simulink model "smm_with_grf_tilting_2d"  (R2014b)
settings: Solver=FixedStepDiscrete  StartTime=0.0  StopTime=inf  FixedStep=sample_time  RelTol=1e-3
undefined symbols (not defined in the file or in its folder): A_lpf_dtau, A_lpf_leg_spring, alpha_apex, alpha_max, alpha_min, B1_lpf_dtau, B1_lpf_leg_spring, B2_lpf_dtau, B2_lpf_leg_spring, boom_mount_angle, boom_pelvis_offset_angle, c_energy, contact_threshold, control_start_time, d_y_boom_com_offset, d_y_boom_hip_offset, d_y_com, desired_torso_angle, dx_avg_desired, enable_torso_wave, fcut_contact, ff_energy_l, ff_energy_r, g, g_reduced, h_boom, HIP_MTR_MAX_CONT_TORQUE, i_robot, initial_com_height, initial_dx, j_leg, j_motor, j_rotor, j_segments, k0_virtual, k_placement, k_sea, kd_lateral, kd_motor, kd_torso, kp_lateral, kp_motor, kp_raibert, kp_torso, l0_leg, l0_min_flight_time, l0_virtual, l0_virtual_raibert, l_boom_projected, l_max, l_retract_delta, l_retract_swing_max, l_retract_swing_min, l_seg, l_yaw_center_to_pelvis, lambda1, lambda2, lateral_offset, lateral_target_angle_left, lateral_target_angle_right ... (+40)
libraries: simulink x24, slrtlib x4, simulink_extras x2
(part 3 of 4)

== system smm_with_grf_tilting_2d/Control/Behavior Control/Primary Leg Behavior/SMM 01/Primary Swing Phase/Back//Front Motor PD ==
  Desired Position [rad] [back front] : Inport
  Desired Velocity [rad/s] [back front] : Inport  Port=2
  Desired Acceleration [rad/s^2] [back front] : Inport  Port=3
  Measured Position [rad] [back front] : Inport  Port=4
  Measured Velocity [rad/s] [back front] : Inport  Port=5
  Right/Left Leg [1/0] : Inport  Port=6
  Friction Compensation : Subsystem
  Product : Product
  Sum1 : Sum  Inputs=|++
  Sum2 : Sum  Inputs=|++
  Sum7 : Sum  Inputs=|+-
  Sum8 : Sum  Inputs=|+-
  Sum9 : Sum
  Switch : Switch  Criteria=u2 ~= 0
  kd : Gain  Gain=kd_motor
  kp : Gain  Gain=kp_motor
  left_inertias : Constant  Value=j_segments(3:4)
  right_inertias : Constant  Value=j_segments(1:2)
  Commanded Torque [Nm] [back front] : Outport
  wires:
  kp/1 -> Sum9/1
  Sum7/1 -> kp/1
  Measured Position [rad] [back front]/1 -> Sum7/2
  Sum9/1 -> Sum1/1
  Sum8/1 -> kd/1
  Desired Position [rad] [back front]/1 -> Sum7/1
  kd/1 -> Sum9/2
  Measured Velocity [rad/s] [back front]/1 -> Sum8/2
  Sum1/1 -> Sum2/1
  Desired Acceleration [rad/s^2] [back front]/1 -> Product/1
  Product/1 -> Sum1/2
  Right/Left Leg [1/0]/1 -> Friction Compensation/1(Right/Left [1/0]), Switch/2
  right_inertias/1 -> Switch/1
  left_inertias/1 -> Switch/3
  Switch/1 -> Product/2
  Sum2/1 -> Commanded Torque [Nm] [back front]/1
  Friction Compensation/1(Friction Compensation [Nm]) -> Sum2/2
  Desired Velocity [rad/s] [back front]/1 -> Friction Compensation/2(Commanded Velocity [rad/s] [back front]), Sum8/1

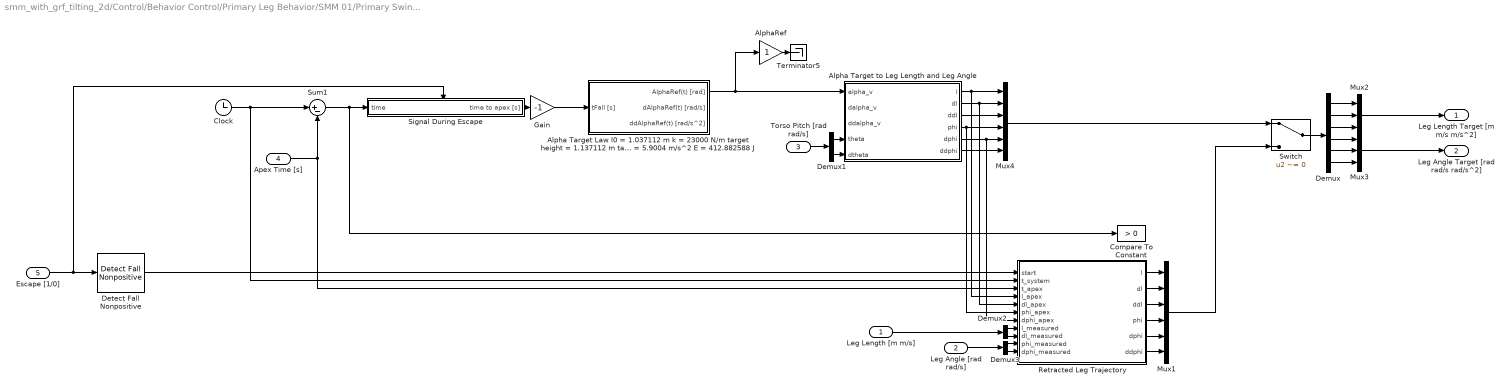
== system smm_with_grf_tilting_2d/Control/Behavior Control/Primary Leg Behavior/SMM 01/Primary Swing Phase/Leg Trajectory Generator (Level Ground) ==
  Leg Length [m m/s] : Inport
  Leg Angle [rad rad/s] : Inport  Port=2
  Torso Pitch [rad rad/s] : Inport  Port=3
  Apex Time [s] : Inport  Port=4
  Escape [1/0] : Inport  Port=5
  Alpha Target Law l0 = 1.037112 m k = 23000 N/m target height = 1.137112 m target speed = 0.5 m/s m = 60.4120 kg g = 5.9004 m/s^2 E = 412.882588 J : Subsystem
  Alpha Target to Leg Length and Leg Angle : MATLAB Function  TreatAsAtomicUnit=on
  AlphaRef : Gain
  Clock : Clock
  Compare To Constant : simulink/Logic and Bit Operations/Compare To Constant  relop=>  const=0  OutDataTypeStr=boolean  ZeroCross=off
  Demux : Demux  Outputs=6
  Demux1 : Demux  Outputs=2
  Demux2 : Demux  Outputs=2
  Demux3 : Demux  Outputs=2
  Detect Fall Nonpositive : simulink/Logic and Bit Operations/Detect Fall Nonpositive  vinit=0  InputProcessing=Inherited  OutDataTypeStr=boolean
  Gain : Gain  Gain=-1
  Mux1 : Mux  Inputs=6
  Mux2 : Mux  Inputs=3
  Mux3 : Mux  Inputs=3
  Mux4 : Mux  Inputs=6
  Retracted Leg Trajectory : MATLAB Function  TreatAsAtomicUnit=on
  Signal During Escape : Subsystem
  Sum1 : Sum  Inputs=|+-
  Switch : Switch  Criteria=u2 ~= 0
  Terminator5 : Terminator
  Leg Length Target [m m/s m/s^2] : Outport
  Leg Angle Target [rad rad/s rad/s^2] : Outport  Port=2
  wires:
  Gain/1 -> Alpha Target Law l0 = 1.037112 m k = 23000 N/m target height = 1.137112 m target speed = 0.5 m/s m = 60.4120 kg g = 5.9004 m/s^2 E = 412.882588 J/1(tFall [s])
  Signal During Escape/1(time to apex [s]) -> Gain/1
  Leg Length [m m/s]/1 -> Demux2/1
  Leg Angle [rad rad/s]/1 -> Demux3/1
  Demux3/2 -> Retracted Leg Trajectory/11(dphi_measured)
  Demux3/1 -> Retracted Leg Trajectory/10(phi_measured)
  Demux2/2 -> Retracted Leg Trajectory/9(dl_measured)
  Demux2/1 -> Retracted Leg Trajectory/8(l_measured)
  Retracted Leg Trajectory/6(ddphi) -> Mux1/6
  Retracted Leg Trajectory/3(ddl) -> Mux1/3
  Mux4/1 -> Switch/1
  Demux1/2 -> Alpha Target to Leg Length and Leg Angle/5(dtheta)
  Demux1/1 -> Alpha Target to Leg Length and Leg Angle/4(theta)
  Demux/1 -> Mux2/1
  Demux/2 -> Mux2/2
  Demux/3 -> Mux2/3
  Demux/4 -> Mux3/1
  Demux/5 -> Mux3/2
  Demux/6 -> Mux3/3
  Mux3/1 -> Leg Angle Target [rad rad/s rad/s^2]/1
  Mux2/1 -> Leg Length Target [m m/s m/s^2]/1
  Switch/1 -> Demux/1
  Alpha Target to Leg Length and Leg Angle/1(l) -> Mux4/1, Retracted Leg Trajectory/4(l_apex)
  Alpha Target to Leg Length and Leg Angle/2(dl) -> Mux4/2, Retracted Leg Trajectory/5(dl_apex)
  Alpha Target to Leg Length and Leg Angle/6(ddphi) -> Mux4/6
  Alpha Target to Leg Length and Leg Angle/5(dphi) -> Mux4/5, Retracted Leg Trajectory/7(dphi_apex)
  Alpha Target to Leg Length and Leg Angle/3(ddl) -> Mux4/3
  Alpha Target to Leg Length and Leg Angle/4(phi) -> Mux4/4, Retracted Leg Trajectory/6(phi_apex)
  Detect Fall Nonpositive/1 -> Retracted Leg Trajectory/1(start)
  Escape [1/0]/1 -> Signal During Escape/Enable, Detect Fall Nonpositive/1
  Retracted Leg Trajectory/5(dphi) -> Mux1/5
  Retracted Leg Trajectory/2(dl) -> Mux1/2
  Retracted Leg Trajectory/4(phi) -> Mux1/4
  Retracted Leg Trajectory/1(l) -> Mux1/1
  AlphaRef/1 -> Terminator5/1
  Sum1/1 -> Compare To Constant/1, Signal During Escape/1(time)
  Alpha Target Law l0 = 1.037112 m k = 23000 N/m target height = 1.137112 m target speed = 0.5 m/s m = 60.4120 kg g = 5.9004 m/s^2 E = 412.882588 J/1(AlphaRef(t) [rad]) -> Alpha Target to Leg Length and Leg Angle/1(alpha_v), AlphaRef/1
  Clock/1 -> Sum1/1, Retracted Leg Trajectory/2(t_system)
  Apex Time [s]/1 -> Sum1/2, Retracted Leg Trajectory/3(t_apex)
  Mux1/1 -> Switch/3
  Torso Pitch [rad rad/s]/1 -> Demux1/1

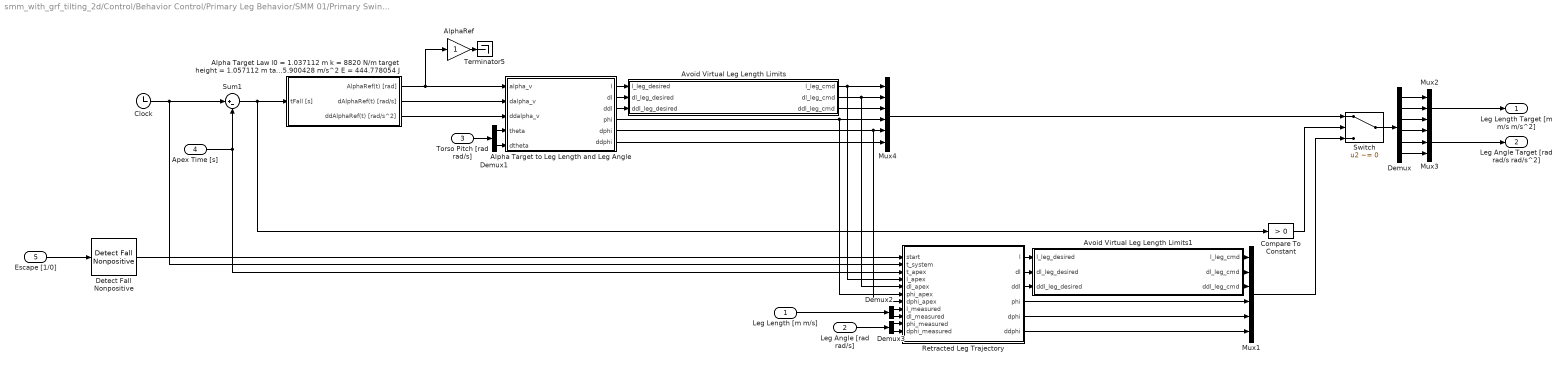
== system smm_with_grf_tilting_2d/Control/Behavior Control/Primary Leg Behavior/SMM 01/Primary Swing Phase/Leg Trajectory Generator (Normal) ==
  Leg Length [m m/s] : Inport
  Leg Angle [rad rad/s] : Inport  Port=2
  Torso Pitch [rad rad/s] : Inport  Port=3
  Apex Time [s] : Inport  Port=4
  Escape [1/0] : Inport  Port=5
  Alpha Target Law l0 = 1.037112 m k = 8820 N/m target height = 1.057112 m target speed = 1.0 m/s m = 60.4120 kg g = 5.900428 m/s^2 E = 444.778054 J : Subsystem
  Alpha Target to Leg Length and Leg Angle : MATLAB Function  TreatAsAtomicUnit=on
  AlphaRef : Gain
  Avoid Virtual Leg Length Limits : MATLAB Function  TreatAsAtomicUnit=on
  Avoid Virtual Leg Length Limits1 : MATLAB Function  TreatAsAtomicUnit=on
  Clock : Clock
  Compare To Constant : simulink/Logic and Bit Operations/Compare To Constant  relop=>  const=0  OutDataTypeStr=boolean  ZeroCross=off
  Demux : Demux  Outputs=6
  Demux1 : Demux  Outputs=2
  Demux2 : Demux  Outputs=2
  Demux3 : Demux  Outputs=2
  Detect Fall Nonpositive : simulink/Logic and Bit Operations/Detect Fall Nonpositive  vinit=0  InputProcessing=Inherited  OutDataTypeStr=boolean
  Mux1 : Mux  Inputs=6
  Mux2 : Mux  Inputs=3
  Mux3 : Mux  Inputs=3
  Mux4 : Mux  Inputs=6
  Retracted Leg Trajectory : MATLAB Function  TreatAsAtomicUnit=on
  Sum1 : Sum  Inputs=|+-
  Switch : Switch  Criteria=u2 ~= 0
  Terminator5 : Terminator
  Leg Length Target [m m/s m/s^2] : Outport
  Leg Angle Target [rad rad/s rad/s^2] : Outport  Port=2
  wires:
  Retracted Leg Trajectory/3(ddl) -> Avoid Virtual Leg Length Limits1/3(ddl_leg_desired)
  Retracted Leg Trajectory/2(dl) -> Avoid Virtual Leg Length Limits1/2(dl_leg_desired)
  Retracted Leg Trajectory/1(l) -> Avoid Virtual Leg Length Limits1/1(l_leg_desired)
  Avoid Virtual Leg Length Limits1/3(ddl_leg_cmd) -> Mux1/3
  Avoid Virtual Leg Length Limits1/2(dl_leg_cmd) -> Mux1/2
  Avoid Virtual Leg Length Limits1/1(l_leg_cmd) -> Mux1/1
  Alpha Target to Leg Length and Leg Angle/3(ddl) -> Avoid Virtual Leg Length Limits/3(ddl_leg_desired)
  Alpha Target to Leg Length and Leg Angle/2(dl) -> Avoid Virtual Leg Length Limits/2(dl_leg_desired)
  Alpha Target to Leg Length and Leg Angle/1(l) -> Avoid Virtual Leg Length Limits/1(l_leg_desired)
  Escape [1/0]/1 -> Detect Fall Nonpositive/1
  Torso Pitch [rad rad/s]/1 -> Demux1/1
  Mux1/1 -> Switch/3
  Compare To Constant/1 -> Switch/2
  Apex Time [s]/1 -> Sum1/2, Retracted Leg Trajectory/3(t_apex)
  Clock/1 -> Sum1/1, Retracted Leg Trajectory/2(t_system)
  Alpha Target Law l0 = 1.037112 m k = 8820 N/m target height = 1.057112 m target speed = 1.0 m/s m = 60.4120 kg g = 5.900428 m/s^2 E = 444.778054 J/1(AlphaRef(t) [rad]) -> AlphaRef/1, Alpha Target to Leg Length and Leg Angle/1(alpha_v)
  Sum1/1 -> Alpha Target Law l0 = 1.037112 m k = 8820 N/m target height = 1.057112 m target speed = 1.0 m/s m = 60.4120 kg g = 5.900428 m/s^2 E = 444.778054 J/1(tFall [s]), Compare To Constant/1
  AlphaRef/1 -> Terminator5/1
  Retracted Leg Trajectory/4(phi) -> Mux1/4
  Retracted Leg Trajectory/5(dphi) -> Mux1/5
  Detect Fall Nonpositive/1 -> Retracted Leg Trajectory/1(start)
  Alpha Target to Leg Length and Leg Angle/4(phi) -> Mux4/4, Retracted Leg Trajectory/6(phi_apex)
  Avoid Virtual Leg Length Limits/3(ddl_leg_cmd) -> Mux4/3
  Alpha Target to Leg Length and Leg Angle/5(dphi) -> Mux4/5, Retracted Leg Trajectory/7(dphi_apex)
  Alpha Target to Leg Length and Leg Angle/6(ddphi) -> Mux4/6
  Avoid Virtual Leg Length Limits/2(dl_leg_cmd) -> Mux4/2, Retracted Leg Trajectory/5(dl_apex)
  Avoid Virtual Leg Length Limits/1(l_leg_cmd) -> Mux4/1, Retracted Leg Trajectory/4(l_apex)
  Switch/1 -> Demux/1
  Mux2/1 -> Leg Length Target [m m/s m/s^2]/1
  Mux3/1 -> Leg Angle Target [rad rad/s rad/s^2]/1
  Demux/6 -> Mux3/3
  Demux/5 -> Mux3/2
  Demux/4 -> Mux3/1
  Demux/3 -> Mux2/3
  Demux/2 -> Mux2/2
  Demux/1 -> Mux2/1
  Demux1/1 -> Alpha Target to Leg Length and Leg Angle/4(theta)
  Demux1/2 -> Alpha Target to Leg Length and Leg Angle/5(dtheta)
  Mux4/1 -> Switch/1
  Alpha Target Law l0 = 1.037112 m k = 8820 N/m target height = 1.057112 m target speed = 1.0 m/s m = 60.4120 kg g = 5.900428 m/s^2 E = 444.778054 J/3(ddAlphaRef(t) [rad/s^2]) -> Alpha Target to Leg Length and Leg Angle/3(ddalpha_v)
  Alpha Target Law l0 = 1.037112 m k = 8820 N/m target height = 1.057112 m target speed = 1.0 m/s m = 60.4120 kg g = 5.900428 m/s^2 E = 444.778054 J/2(dAlphaRef(t) [rad/s]) -> Alpha Target to Leg Length and Leg Angle/2(dalpha_v)
  Retracted Leg Trajectory/6(ddphi) -> Mux1/6
  Demux2/1 -> Retracted Leg Trajectory/8(l_measured)
  Demux2/2 -> Retracted Leg Trajectory/9(dl_measured)
  Demux3/1 -> Retracted Leg Trajectory/10(phi_measured)
  Demux3/2 -> Retracted Leg Trajectory/11(dphi_measured)
  Leg Angle [rad rad/s]/1 -> Demux3/1
  Leg Length [m m/s]/1 -> Demux2/1

== system smm_with_grf_tilting_2d/Control/Behavior Control/Primary Leg Behavior/Raibert Hopping/Inverse Dynamics Virtual Spring/Angle Sine Wave/Timer ==
  Enable : EnablePort  StatesWhenEnabling=reset  ShowOutputPort=on
  Constant : Constant
  Discrete-Time Integrator : DiscreteIntegrator  IntegratorMethod=Accumulation: Forward Euler  gainval=sample_time  ExternalReset=rising  SampleTime=sample_time
  timer [s] : Outport  InitialOutput=[0]
  wires:
  Discrete-Time Integrator/1 -> timer [s]/1
  Enable/1 -> Discrete-Time Integrator/2
  Constant/1 -> Discrete-Time Integrator/1

== system smm_with_grf_tilting_2d/Control/Behavior Control/Primary Leg Behavior/Raibert Hopping/Spring Rest Length/Hold Initial/Subsystem ==
  in : Inport
  Enable : EnablePort
  out : Outport  InitialOutput=[l0_virtual_raibert]
  wires:
  in/1 -> out/1

== system smm_with_grf_tilting_2d/Control/Behavior Control/Primary Leg Behavior/SMM 01/Primary Stance Phase/Virtual Leg Force and Swing Leg Retraction/Hold Initial ==
  in : Inport
  Trigger : TriggerPort  ShowOutputPort=on  PortDimensions=1
  Subsystem : Subsystem
  out : Outport  InitialOutput=[l0_virtual]
  wires:
  Trigger/1 -> Subsystem/Enable
  Subsystem/1(out) -> out/1
  in/1 -> Subsystem/1(in)

== system smm_with_grf_tilting_2d/Control/Behavior Control/Primary Leg Behavior/SMM 01/Primary Stance Phase/Virtual Leg Force and Swing Leg Retraction/Leg Force-Torque Distribution ==
  Front Spring Torque [Nm] : Inport
  Back Spring Torque [Nm] : Inport  Port=2
  w [m] : Inport  Port=3
  Divide : Product  Inputs=*/
  Sum2 : Sum  Inputs=+|+
  Sum5 : Sum  Inputs=+|-
  Leg Force [N] : Outport
  Leg Torque [Nm] : Outport  Port=2
  wires:
  Sum2/1 -> Leg Torque [Nm]/1
  Back Spring Torque [Nm]/1 -> Sum5/2, Sum2/2
  Sum5/1 -> Divide/1
  w [m]/1 -> Divide/2
  Front Spring Torque [Nm]/1 -> Sum5/1, Sum2/1
  Divide/1 -> Leg Force [N]/1

== system smm_with_grf_tilting_2d/Control/Behavior Control/Primary Leg Behavior/SMM 01/Primary Stance Phase/Virtual Leg Force and Swing Leg Retraction/Touch Down Trigger ==
  Flight [1/0] : Inport
  Compare To Constant : simulink/Logic and Bit Operations/Compare To Constant  relop=>  const=l0_min_flight_time  OutDataTypeStr=boolean
  Data Type Conversion1 : DataTypeConversion  OutDataTypeStr=boolean
  Logical Operator : Logic  Operator=NOT  IconShape=distinctive  AllPortsSameDT=off  OutDataTypeStr=boolean
  Logical Operator4 : Logic  IconShape=distinctive  AllPortsSameDT=off  OutDataTypeStr=boolean
  S-R Flip-Flop : simulink_extras/Flip Flops/S-R Flip-Flop  initial_condition=0
  Timer : Subsystem
  Trigger [1/0] : Outport
  wires:
  Compare To Constant/1 -> Logical Operator4/2
  S-R Flip-Flop/1 -> Trigger [1/0]/1
  Timer/1(timer [s]) -> Compare To Constant/1
  Logical Operator/1 -> Logical Operator4/1
  Logical Operator4/1 -> S-R Flip-Flop/1
  Flight [1/0]/1 -> Data Type Conversion1/1, Timer/Enable, Logical Operator/1
  Data Type Conversion1/1 -> S-R Flip-Flop/2

== system smm_with_grf_tilting_2d/Control/Behavior Control/Primary Leg Behavior/SMM 01/Primary Swing Phase/Back//Front Motor PD/Friction Compensation ==
  Right/Left [1/0] : Inport
  Commanded Velocity [rad/s] [back front] : Inport  Port=2
  Product : Product
  Sign : Signum
  Sum1 : Sum
  Switch : Switch  Criteria=u2 ~= 0
  Switch1 : Switch  Criteria=u2 ~= 0
  coulomb_friction_left : Constant  Value=sea_coulomb_friction(3:4)
  coulomb_friction_right : Constant  Value=sea_coulomb_friction(1:2)
  offset_friction_left : Constant  Value=sea_offset_friction(3:4)
  offset_friction_right : Constant  Value=sea_offset_friction(1:2)
  Friction Compensation [Nm] : Outport
  wires:
  Commanded Velocity [rad/s] [back front]/1 -> Sign/1
  Switch/1 -> Sum1/2
  Sum1/1 -> Friction Compensation [Nm]/1
  Product/1 -> Sum1/1
  Right/Left [1/0]/1 -> Switch1/2, Switch/2
  offset_friction_right/1 -> Switch/1
  offset_friction_left/1 -> Switch/3
  coulomb_friction_right/1 -> Switch1/1
  coulomb_friction_left/1 -> Switch1/3
  Switch1/1 -> Product/2
  Sign/1 -> Product/1

== system smm_with_grf_tilting_2d/Control/Behavior Control/Primary Leg Behavior/SMM 01/Primary Swing Phase/Leg Trajectory Generator (Level Ground)/Alpha Target Law l0 = 1.037112 m k = 23000 N//m target height = 1.137112 m target speed = 0.5 m//s m = 60.4120 kg g = 5.9004 m//s^2 E = 412.882588 J ==
  note: Angle of Attack Control Law From Poincare Map Method
  tFall [s] : Inport
  Alpha Target Polynomials : Subsystem
  AlphaRef1 : Constant  Value=[(90+20)*pi/180 0 0]
  Compare To Constant1 : simulink/Logic and Bit Operations/Compare To Constant  relop=<  const=0.19512514  OutDataTypeStr=boolean  ZeroCross=off
  Demux : Demux  Outputs=3
  Ignore Negatives : Fcn  Expr=(u >= 0)*u
  Mux : Mux  Inputs=3
  Switch : Switch  Criteria=u2 ~= 0
  AlphaRef(t) [rad] : Outport
  dAlphaRef(t) [rad/s] : Outport  Port=2
  ddAlphaRef(t) [rad/s^2] : Outport  Port=3
  wires:
  Ignore Negatives/1 -> Alpha Target Polynomials/1(tFall)
  Mux/1 -> Switch/1
  Alpha Target Polynomials/1(AlphaRef(t)) -> Mux/1
  Alpha Target Polynomials/3(ddAlphaRef(t)) -> Mux/3
  Alpha Target Polynomials/2(dAlphaRef(t)) -> Mux/2
  Compare To Constant1/1 -> Switch/2
  tFall [s]/1 -> Compare To Constant1/1, Ignore Negatives/1
  Switch/1 -> Demux/1
  Demux/1 -> AlphaRef(t) [rad]/1
  Demux/2 -> dAlphaRef(t) [rad/s]/1
  Demux/3 -> ddAlphaRef(t) [rad/s^2]/1
  AlphaRef1/1 -> Switch/3

== system smm_with_grf_tilting_2d/Control/Behavior Control/Primary Leg Behavior/SMM 01/Primary Swing Phase/Leg Trajectory Generator (Level Ground)/Signal During Escape ==
  time : Inport
  Enable : EnablePort
  time to apex [s] : Outport
  wires:
  time/1 -> time to apex [s]/1

== system smm_with_grf_tilting_2d/Control/Behavior Control/Primary Leg Behavior/SMM 01/Primary Swing Phase/Leg Trajectory Generator (Normal)/Alpha Target Law l0 = 1.037112 m k = 8820 N//m target height = 1.057112 m target speed = 1.0 m//s m = 60.4120 kg g = 5.900428 m//s^2 E = 444.778054 J ==
  note: Angle of Attack Control Law From Poincare Map Method
  tFall [s] : Inport
  Alpha Target Polynomials : Subsystem
  AlphaRef1 : Constant  Value=[(90+20)*pi/180 0 0]
  Compare To Constant1 : simulink/Logic and Bit Operations/Compare To Constant  relop=<  const=0.33124891  OutDataTypeStr=boolean  ZeroCross=off
  Demux : Demux  Outputs=3
  Ignore Negatives : Fcn  Expr=(u >= 0)*u
  Mux : Mux  Inputs=3
  Switch : Switch  Criteria=u2 ~= 0
  AlphaRef(t) [rad] : Outport
  dAlphaRef(t) [rad/s] : Outport  Port=2
  ddAlphaRef(t) [rad/s^2] : Outport  Port=3
  wires:
  Alpha Target Polynomials/1(AlphaRef(t)) -> Mux/1
  AlphaRef1/1 -> Switch/3
  Demux/3 -> ddAlphaRef(t) [rad/s^2]/1
  Demux/2 -> dAlphaRef(t) [rad/s]/1
  Demux/1 -> AlphaRef(t) [rad]/1
  Switch/1 -> Demux/1
  tFall [s]/1 -> Ignore Negatives/1, Compare To Constant1/1
  Compare To Constant1/1 -> Switch/2
  Alpha Target Polynomials/2(dAlphaRef(t)) -> Mux/2
  Alpha Target Polynomials/3(ddAlphaRef(t)) -> Mux/3
  Mux/1 -> Switch/1
  Ignore Negatives/1 -> Alpha Target Polynomials/1(tFall)

== system smm_with_grf_tilting_2d/Control/Behavior Control/Primary Leg Behavior/SMM 01/Primary Stance Phase/Virtual Leg Force and Swing Leg Retraction/Hold Initial/Subsystem ==
  in : Inport
  Enable : EnablePort
  out : Outport  InitialOutput=[l0_virtual]
  wires:
  in/1 -> out/1

== system smm_with_grf_tilting_2d/Control/Behavior Control/Primary Leg Behavior/SMM 01/Primary Stance Phase/Virtual Leg Force and Swing Leg Retraction/Touch Down Trigger/Timer ==
  Enable : EnablePort  StatesWhenEnabling=reset  ShowOutputPort=on
  Constant : Constant
  Discrete-Time Integrator : DiscreteIntegrator  IntegratorMethod=Accumulation: Forward Euler  gainval=sample_time  ExternalReset=rising  SampleTime=sample_time
  timer [s] : Outport  InitialOutput=[0]
  wires:
  Discrete-Time Integrator/1 -> timer [s]/1
  Enable/1 -> Discrete-Time Integrator/2
  Constant/1 -> Discrete-Time Integrator/1

== system smm_with_grf_tilting_2d/Control/Behavior Control/Primary Leg Behavior/SMM 01/Primary Swing Phase/Leg Trajectory Generator (Level Ground)/Alpha Target Law l0 = 1.037112 m k = 23000 N//m target height = 1.137112 m target speed = 0.5 m//s m = 60.4120 kg g = 5.9004 m//s^2 E = 412.882588 J/Alpha Target Polynomials ==
  tFall : Inport
  AlphaRef(t) Control Law : Fcn  Expr=1.0339*u^3 + 6.848*u^2 + 3.5731*u + alpha_apex
  acceleration of AlphaRef(t) Control Law : Fcn  Expr=2*3*1.0339*u + 2*6.848
  velocity of AlphaRef(t) Control Law : Fcn  Expr=3*1.0339*u^2 + 2*6.848*u + 3.5731
  AlphaRef(t) : Outport  OutputWhenDisabled=reset  InitialOutput=0
      settings: AttributesFormatString=When disabled: %<OutputWhenDisabled>\nDisabled Output: %<InitialOutput>
  dAlphaRef(t) : Outport  Port=2  OutputWhenDisabled=reset  InitialOutput=0
      settings: AttributesFormatString=When disbaled: %<OutputWhenDisabled>\nDisabled output: %<InitialOutput>
  ddAlphaRef(t) : Outport  Port=3  OutputWhenDisabled=reset  InitialOutput=0
      settings: AttributesFormatString=When disabled: %<OutputWhenDisabled>\nDisabled output: %<InitialOutput>
  wires:
  tFall/1 -> AlphaRef(t) Control Law/1, velocity of AlphaRef(t) Control Law/1, acceleration of AlphaRef(t) Control Law/1
  AlphaRef(t) Control Law/1 -> AlphaRef(t)/1
  velocity of AlphaRef(t) Control Law/1 -> dAlphaRef(t)/1
  acceleration of AlphaRef(t) Control Law/1 -> ddAlphaRef(t)/1

== system smm_with_grf_tilting_2d/Control/Behavior Control/Primary Leg Behavior/SMM 01/Primary Swing Phase/Leg Trajectory Generator (Normal)/Alpha Target Law l0 = 1.037112 m k = 8820 N//m target height = 1.057112 m target speed = 1.0 m//s m = 60.4120 kg g = 5.900428 m//s^2 E = 444.778054 J/Alpha Target Polynomials ==
  tFall : Inport
  AlphaRef(t) Control Law : Fcn  Expr=12.835*u^3 - 2.9736*u^2 + 1.9343*u + alpha_apex
  acceleration of AlphaRef(t) Control Law : Fcn  Expr=2*3*12.835*u - 2*2.9736
  velocity of AlphaRef(t) Control Law : Fcn  Expr=3*12.835*u^2 - 2*2.9736*u + 1.9343
  AlphaRef(t) : Outport  OutputWhenDisabled=reset  InitialOutput=0
      settings: AttributesFormatString=When disabled: %<OutputWhenDisabled>\nDisabled Output: %<InitialOutput>
  dAlphaRef(t) : Outport  Port=2  OutputWhenDisabled=reset  InitialOutput=0
      settings: AttributesFormatString=When disbaled: %<OutputWhenDisabled>\nDisabled output: %<InitialOutput>
  ddAlphaRef(t) : Outport  Port=3  OutputWhenDisabled=reset  InitialOutput=0
      settings: AttributesFormatString=When disabled: %<OutputWhenDisabled>\nDisabled output: %<InitialOutput>
  wires:
  acceleration of AlphaRef(t) Control Law/1 -> ddAlphaRef(t)/1
  velocity of AlphaRef(t) Control Law/1 -> dAlphaRef(t)/1
  AlphaRef(t) Control Law/1 -> AlphaRef(t)/1
  tFall/1 -> acceleration of AlphaRef(t) Control Law/1, velocity of AlphaRef(t) Control Law/1, AlphaRef(t) Control Law/1

== stateflow chart smm_with_grf_tilting_2d/Control/Behavior Control/Primary Leg Behavior/State Machine ==
  state TouchDown
    entry: placement = false;
    entry: posture = false;
    entry: thrust = false;
    entry: flight = false;
    entry: escape = false;
  state LockedContact
    entry: placement = false;
    entry: posture = true;
    entry: thrust = false;
    entry: flight = false;
    entry: escape = false;
  state Rebound
    entry: placement = false;
    entry: posture = true;
    entry: thrust = true;
    entry: flight = false;
    entry: escape = false;
  state Unloading
    entry: placement = false;
    entry: posture = false;
    entry: thrust = true;
    entry: flight = false;
    entry: escape = false;
  state TakeOff
    entry: placement = false;
    entry: posture = false;
    entry: thrust = false;
    entry: flight = true;
    entry: escape = true;
  state Flight
    entry: placement = true;
    entry: posture = false;
    entry: thrust = false;
    entry: flight = true;
    entry: escape = false;
  (junction 91) -> TouchDown
  TouchDown -> (junction 130) [order 2] : [Fy < contact_threshold]
  (junction 93) -> (junction 91)
  (junction 130) -> (junction 128)
  TouchDown -> LockedContact [order 1] : [Fy > loaded_threshold]
  (junction 115) -> LockedContact
  (junction 118) -> (junction 115)
  LockedContact -> Rebound : [dl >= 0 && dl_prev < 0]
  Rebound -> Unloading [order 1] : [Fy < loaded_threshold]
  Rebound -> (junction 102) [order 2] : [l > l_max]
  (junction 102) -> (junction 100)
  (junction 122) -> (junction 118)
  Unloading -> TakeOff [order 1] : [Fy < contact_threshold || l > l_max]
  Unloading -> (junction 122) [order 2] : [Fy > loaded_threshold && dl < 0]
  TakeOff -> Flight : after(t_flight,sec)
  (junction 100) -> TakeOff
  (default) -> Flight
  Flight -> (junction 93) : [Fy > contact_threshold]
  (junction 128) -> Flight
  data: flight output; escape output; thrust output; posture output; l input; dl input; dl_prev input; Fy input; t_flight parameter; placement output; l_max parameter; contact_threshold parameter; loaded_threshold parameter

== matlab function smm_with_grf_tilting_2d/Control/Behavior Control/Primary Leg Behavior/SMM 01/Primary Swing Phase/Leg Trajectory Generator (Normal)/Avoid Virtual Leg Length Limits ==
  data: l_leg_desired input; dl_leg_desired input; ddl_leg_desired input; l_leg_cmd output double; dl_leg_cmd output double; ddl_leg_cmd output double; min_leg_length parameter; max_leg_length parameter
%% Avoid virtual leg length limits by ensuring we don't command position/velocities/accelerations that would hit them.
function [l_leg_cmd, dl_leg_cmd, ddl_leg_cmd] = AvoidVirtualLengthLimits(l_leg_desired, dl_leg_desired, ddl_leg_desired, min_leg_length, max_leg_length)
    [l_leg_cmd, dl_leg_cmd, ddl_leg_cmd] = AvoidVirtualLengthLimits(l_leg_desired, dl_leg_desired, ddl_leg_desired, min_leg_length, max_leg_length);
end

== matlab function smm_with_grf_tilting_2d/Control/Behavior Control/Torque Distribution Right/Motor Torque Saturation Optimization ==
  data: x1s input; t1 output; x2s input; lambda1 parameter; lambda2 parameter; max_torque_sagittal parameter; t2 output
% Optimal leg motor torque distribution
function [t1, t2] = distribute_torque(x1s, x2s, lambda1, lambda2, max_torque_sagittal)

s = max_torque_sagittal;

% possible solutions
x1 = [                                                      x1s;
                                                            0;
                                                            s;
                                                            0;
                                                           -s;
  (lambda2*s + lambda1*x1s - lambda2*x2s)/(lambda1 + lambda2);
  (lambda1*x1s - lambda2*s + lambda2*x2s)/(lambda1 + lambda2);
  (lambda2*s + lambda1*x1s + lambda2*x2s)/(lambda1 + lambda2);
 -(lambda2*s - lambda1*x1s + lambda2*x2s)/(lambda1 + lambda2)];
 
x2 = [                                                      x2s;
                                                            s;
                                                            0;
                                                           -s;
                                                            0;
  (lambda1*s - lambda1*x1s + lambda2*x2s)/(lambda1 + lambda2);
  (lambda1*s + lambda1*x1s + lambda2*x2s)/(lambda1 + lambda2);
  (lambda1*x1s - lambda1*s + lambda2*x2s)/(lambda1 + lambda2);
 -(lambda1*s + lambda1*x1s - lambda2*x2s)/(lambda1 + lambda2)];

% test constraints
c1 = s - x1 - x2 >= 0;
c2 = s + x1 + x2 >= 0;
c3 = s - x1 + x2 >= 0;
c4 = s + x1 - x2 >= 0;
constraints = c1 & c2 & c3 & c4;

% objective function to maximize
f = -lambda1*(x1-x1s).^2-lambda2*(x2-x2s).^2;
satisfied = find(constraints);
[~,I] = max(f(satisfied));

t1 = x1(satisfied(I));
t2 = x2(satisfied(I));

== matlab function smm_with_grf_tilting_2d/Control/Behavior Control/Primary Leg Behavior/Raibert Hopping/Calculate Leg Length From Virtual Spring Length ==
  data: phi input; dphi input; ddphi input; l_virtual input; dl_virtual input; ddl_virtual input; l_leg_target output; d_y_com parameter
function l_leg_target  = VirtualSpringLengthToLegLength(phi, dphi, ddphi, l_virtual, dl_virtual, ddl_virtual, d_y_com)
    [l_leg_target, ~, ~] = VirtualSpringLengthToLegLength(phi, dphi, ddphi, l_virtual, dl_virtual, ddl_virtual, d_y_com);
end

== matlab function smm_with_grf_tilting_2d/Control/Behavior Control/Secondary Leg Behavior/Avoid Hitting Mechanical Limits ==
  data: back_cmd output double; front_cmd output double; dback_cmd output double; dfront_cmd output double; ddback_cmd output double; ddfront_cmd output double; back_desired input; dback_desired input; ddback_desired input; front_desired input; dfront_desired input; ddfront_desired input; min_front_bar_angle parameter; max_front_bar_angle parameter; min_back_bar_angle parameter; max_back_bar_angle parameter
%% Avoid joint limits by ensuring we don't command velocities/accelerations that would push us into them when we are close to them.
function [back_cmd, front_cmd, dback_cmd, dfront_cmd, ddback_cmd, ddfront_cmd] ...
    = AvoidFourbarLimits(back_desired,dback_desired, ddback_desired, ...
          front_desired, dfront_desired, ddfront_desired, ...
          min_front_bar_angle, max_front_bar_angle, min_back_bar_angle, max_back_bar_angle)
    [back_cmd, front_cmd, dback_cmd, dfront_cmd, ddback_cmd, ddfront_cmd] = AvoidFourbarLimits(back_desired,dback_desired, ddback_desired, front_desired, dfront_desired, ddfront_desired, min_front_bar_angle, max_front_bar_angle, min_back_bar_angle, max_back_bar_angle);
end

== matlab function smm_with_grf_tilting_2d/Control/Behavior Control/Velocity Estimation/dx_and_dy_from_yaw_and_roll ==
  data: qRoll input; dqRoll input; qYaw input; dx_com output; dqYaw input; qPitch input; dqPitch input; l_boom_projected parameter; h_boom parameter; boom_mount_angle parameter; d_y_boom_com_offset parameter; d_y_boom_hip_offset parameter; dy_com output; x_com output; x_hip output; y_com output; y_hip output
function [dx_com, dy_com, x_com, x_hip, y_com, y_hip] = fcn(qRoll, dqRoll, qYaw, dqYaw, qPitch, dqPitch, ...
                        l_boom_projected, h_boom, boom_mount_angle, ...
                        d_y_boom_com_offset, d_y_boom_hip_offset)

    % y position
    y_com = h_boom + l_boom_projected * sin(qRoll)  -  d_y_boom_com_offset * cos(qRoll-boom_mount_angle) * cos(qPitch);
    y_hip = h_boom + l_boom_projected * sin(qRoll)  -  d_y_boom_hip_offset * cos(qRoll-boom_mount_angle) * cos(qPitch);
    
    % y velocity
    dy_com = l_boom_projected*dqRoll*cos(qRoll) + d_y_boom_com_offset*dqPitch*sin(qPitch)*cos(qRoll - boom_mount_angle) + d_y_boom_com_offset*dqRoll*cos(qPitch)*sin(qRoll - boom_mount_angle);
    
    % x position
    x_com = l_boom_projected * cos(qRoll) * qYaw - d_y_boom_com_offset * sin(qPitch) * cos(qRoll-boom_mount_angle);
    x_hip = l_boom_projected * cos(qRoll) * qYaw - d_y_boom_hip_offset * sin(qPitch) * cos(qRoll-boom_mount_angle);
    
    % x velocity
    dx_com = l_boom_projected*dqYaw*cos(qRoll) - l_boom_projected*dqRoll*sin(qRoll)*qYaw - d_y_boom_com_offset*dqPitch*cos(qPitch)*cos(qRoll - boom_mount_angle) + d_y_boom_com_offset*dqRoll*sin(qPitch)*sin(qRoll - boom_mount_angle);
 
    
end

== matlab function smm_with_grf_tilting_2d/Control/Behavior Control/Torque Distribution Left/Motor Torque Saturation Optimization ==
  data: x1s input; t1 output; x2s input; lambda1 parameter; lambda2 parameter; max_torque_sagittal parameter; t2 output
% Optimal leg motor torque distribution
function [t1, t2] = distribute_torque(x1s, x2s, lambda1, lambda2, max_torque_sagittal)

s = max_torque_sagittal;

% possible solutions
x1 = [                                                      x1s;
                                                            0;
                                                            s;
                                                            0;
                                                           -s;
  (lambda2*s + lambda1*x1s - lambda2*x2s)/(lambda1 + lambda2);
  (lambda1*x1s - lambda2*s + lambda2*x2s)/(lambda1 + lambda2);
  (lambda2*s + lambda1*x1s + lambda2*x2s)/(lambda1 + lambda2);
 -(lambda2*s - lambda1*x1s + lambda2*x2s)/(lambda1 + lambda2)];
 
x2 = [                                                      x2s;
                                                            s;
                                                            0;
                                                           -s;
                                                            0;
  (lambda1*s - lambda1*x1s + lambda2*x2s)/(lambda1 + lambda2);
  (lambda1*s + lambda1*x1s + lambda2*x2s)/(lambda1 + lambda2);
  (lambda1*x1s - lambda1*s + lambda2*x2s)/(lambda1 + lambda2);
 -(lambda1*s + lambda1*x1s - lambda2*x2s)/(lambda1 + lambda2)];

% test constraints
c1 = s - x1 - x2 >= 0;
c2 = s + x1 + x2 >= 0;
c3 = s - x1 + x2 >= 0;
c4 = s + x1 - x2 >= 0;
constraints = c1 & c2 & c3 & c4;

% objective function to maximize
f = -lambda1*(x1-x1s).^2-lambda2*(x2-x2s).^2;
satisfied = find(constraints);
[~,I] = max(f(satisfied));

t1 = x1(satisfied(I));
t2 = x2(satisfied(I));

== matlab function smm_with_grf_tilting_2d/Control/Behavior Control/Velocity Estimation/Takeoff Velocity/vertical_velocity ==
  data: y output; dx output; dy output double; l input; dl input; phi input; dphi input; qPitch input; dqPitch input; d_y_com parameter
function [y,dx,dy] = fcn(l, dl, phi, dphi, qPitch, dqPitch, d_y_com)

% y = -l*cos(theta+phi) + d*cos(theta)
% dy = -dl*cos(theta+phi) + l*(dtheta+dphi)*sin(theta+phi) - d*dtheta*sin(theta)
gamma = phi + qPitch;
dgamma = dphi + dqPitch;
d = d_y_com;

y = -l*cos(gamma) + d*cos(qPitch);
dy = -dl*cos(gamma) + l*dgamma*sin(gamma) - d*dqPitch*sin(qPitch);

% x = -l*sin(gamma) + d*sin(theta)
% dx = -dl*sin(gamma) - l*dgamma*cos(gamma) + d*dtheta*cos(theta)

dx = -dl*sin(gamma) - l*dgamma*cos(gamma) + d*dqPitch*cos(qPitch);

== matlab function smm_with_grf_tilting_2d/Control/Behavior Control/Primary Leg Behavior/SMM 01/Primary Stance Phase/Virtual Leg Force and Swing Leg Retraction/target_GRF_inverse_dynamics ==
  data: z output; k_virtual input; l_virtual input; theta input; phi input; l_leg input; w input; tau_rotor_f input; tau_rotor_b input; d_y_com parameter; l0_virtual parameter; LEG_MTR_GEAR_RATIO parameter; g_reduced parameter; j_leg parameter; j_rotor parameter; i_robot parameter; m_total_real parameter; m_boom parameter; m_leg parameter; GRFx output; GRFy output; kp_torso parameter; kd_torso parameter; desired_torso_angle parameter; GRF_angle output; max_GRF_angle parameter
%% Inverse dynamics
% Inputs:  gamma, dgamma, theta, dtheta,  GRFx_des, GRFy_des
% Outputs: ddx,   ddy,    ddl,   ddgamma, ddtheta,  tau_sf,  tau_sb
function [z, GRFx, GRFy, GRF_angle]  = fcn(k_virtual, l_virtual, theta, phi, l_leg, w,...
                  tau_rotor_f, tau_rotor_b, ...
                  d_y_com, l0_virtual, LEG_MTR_GEAR_RATIO, g_reduced,...
                  j_leg, j_rotor, i_robot, ...
                  m_total_real, m_boom, m_leg, ...
                  kp_torso, kd_torso, desired_torso_angle, max_GRF_angle)

              
              
    % Parameters
    m      = m_total_real;    % mass of system + boom
    Il     = j_leg;             % inertia of leg
    Ir     = j_rotor;           % inertia of rotor
    It     = i_robot;           % inertia of system
    d      = d_y_com;             % distance from hip to system COM
    g1     = phi(1)+theta(1);   % global leg angle (after spring)
    dg1    = phi(2)+theta(2);
    th     = theta(1);          % global torso angle   
    dth    = theta(2);
    t_rf   = tau_rotor_f;       % torque applied at front rotor 
    t_rb   = tau_rotor_b;       % torque applied at back rotor
    N      = -LEG_MTR_GEAR_RATIO;
    l      = l_leg(1);          % leg length
    dl     = l_leg(2);
    lv     = l_virtual(1);      % virtual spring length
    dx     = -l*dg1*cos(g1)+dth*cos(th);
    dy     = l*dg1*sin(g1)-dth*sin(th);
    
    
    
    % Target GRFs
    delta_lv = l0_virtual -  lv;
    GRF = k_virtual*delta_lv* ...
                        [(d*sin(th)-l*sin(g1))/lv; ...
                         (d*cos(th)-l*cos(g1))/lv];
    GRF_angle = atan2(GRF(2),GRF(1));
                     
                     
                     
    % Trunk posture correction 
    F_reg = 1; % prevent division by zero
    ddth_desired = kp_torso*(desired_torso_angle - th) - kd_torso*dth; % PD law
    sine_ratio = It*ddth_desired / (lv*(norm(GRF) + F_reg));
    max_angle = 20*pi/180;
    sine_ratio = min(sin(max_angle), max(-sin(max_angle), sine_ratio));  % saturate rotation angle
    GRF_rotation = asin(sine_ratio);
    GRF_full_angle = GRF_rotation + GRF_angle; % saturate GRF angle
    if GRF_full_angle > (pi-max_GRF_angle)
        GRF_rotation = (pi-max_GRF_angle) - GRF_angle;
    elseif GRF_full_angle < max_GRF_angle
        GRF_rotation = max_GRF_angle - GRF_angle;  
    end
    R = [cos(GRF_rotation)  -sin(GRF_rotation); sin(GRF_rotation) cos(GRF_rotation)];
    GRF_target = R*GRF; % rotate GRF CCW
    GRFx = GRF_target(1);
    GRFy = GRF_target(2);
    GRF_angle = atan2(GRFy,GRFx);
    
    
    
    
    % Stance dynamics (P z = [h; -dJ*dq] + [J zeros(2,2)]^T F)
    %     J  = [1  0  sin(g1)     l*cos(g1)   -d*cos(th);
    %           0  1  cos(g1)    -l*sin(g1)    d*sin(th)];
    %       
    %     dJ = [0  0   dg1*cos(g1)    (-l*dg1*sin(g1)+dl*cos(g1))  d*dth*sin(th);
    %           0  0  -dg1*sin(g1)    (-1*dg1*cos(g1)-dl*sin(g1))  d*dth*cos(th)];
    % 
    %     dq  = [dx  dy  dl  dg1  dth ]';
    %       
    %     M = [m  0   0       0    0; 
    %          0  m   0       0    0;
    %          0  0   m_leg   0    0;   
    %          0  0   0       Il   0;  
    %          0  0   0       0    It];  
    %     
    %     h = [0; -m*g_reduced; 0; 0; (-t_rf-t_rb)];
    % 
    %     S = [ 0         0;
    %           0         0;
    %           1/w      -1/w;
    %           1         1;
    %          -(N-1)/N  -(N-1)/N];
    % 
    %     F = [GRFx GRFy]';
    %     
    %     P = [M              -S;       
    %          J               zeros(2,2)];
    
    % Solving for z:    
    %     ddq = [ddx ddy ddl ddg1 ddth]';
    %     z = [ddq; t_sf; t_sb];
    %     z = P\([h; -dJ*dq] + [J zeros(2,2)]'*F);
    
    z =  [GRFx/m;
         (GRFy - g_reduced*m)/m;
        -(Il*d*dg1^2*m*cos(g1 - th) - 2*GRFx*Il*d*sin(th) - 2*Il*d^2*dth^2*m - GRFy*d*l^2*m*cos(th) - GRFx*d*l^2*m*sin(th) - 2*GRFy*Il*d*cos(th) + 2*GRFy*It*N*l*cos(g1) + 2*GRFy*Il*N*d*cos(th) + 2*GRFx*It*N*l*sin(g1) + 2*GRFx*Il*N*d*sin(th) - It*N*dg1^2*l*m + GRFy*d*l^2*m*cos(2*g1 - th) + GRFx*d*l^2*m*sin(2*g1 - th) + 2*Il*d*g_reduced*m*cos(th) + Il*d*dg1^2*m*cos(g1 + th) + 2*Il*N*d^2*dth^2*m - It*N*dg1^2*l^2*m - 2*It*N*g_reduced*l*m*cos(g1) - 2*Il*N*d*g_reduced*m*cos(th) + It*N*dg1^2*l^2*m*cos(2*g1) - Il*N*d*dg1^2*m*cos(g1 + th) - Il*d*dg1^2*l*m*cos(g1 + th) + 4*Il*d*dg1*dl*m*sin(g1 - th) + GRFy*N*d^2*l*m*cos(g1) + GRFy*N*d*l^2*m*cos(th) + GRFx*N*d^2*l*m*sin(g1) + 2*N*d*l*m*t_rb*sin(g1 - th) + 2*N*d*l*m*t_rf*sin(g1 - th) + GRFx*N*d*l^2*m*sin(th) - Il*N*d*dg1^2*m*cos(g1 - th) - GRFy*N*d^2*l*m*cos(g1 - 2*th) + GRFx*N*d^2*l*m*sin(g1 - 2*th) + Il*d*dg1^2*l*m*cos(g1 - th) - It*N*dg1^2*l*m*cos(2*g1) - GRFy*N*d*l^2*m*cos(2*g1 - th) - GRFx*N*d*l^2*m*sin(2*g1 - th) + Il*N*d*dg1^2*l*m*cos(g1 + th) - 4*Il*N*d*dg1*dl*m*sin(g1 - th) - Il*N*d*dg1^2*l*m*cos(g1 - th) + 2*It*N*d*dth^2*l*m*cos(g1 - th))/(2*m*(It*N*l - Il*d*cos(g1 - th) + Il*N*d*cos(g1 - th)));
        -(2*GRFx*It*N*cos(g1) - 2*GRFy*It*N*sin(g1) + GRFx*N*d^2*m*cos(g1 - 2*th) + 4*It*N*dg1*dl*m + GRFy*N*d^2*m*sin(g1 - 2*th) + GRFx*d*l*m*cos(2*g1 - th) - GRFy*d*l*m*sin(2*g1 - th) + It*N*dg1^2*m*sin(2*g1) + 2*It*N*g_reduced*m*sin(g1) + GRFx*d*l*m*cos(th) - GRFy*d*l*m*sin(th) + GRFx*N*d^2*m*cos(g1) + 2*N*d*m*t_rb*cos(g1 - th) + 2*N*d*m*t_rf*cos(g1 - th) - GRFy*N*d^2*m*sin(g1) - GRFx*N*d*l*m*cos(th) + GRFy*N*d*l*m*sin(th) - GRFx*N*d*l*m*cos(2*g1 - th) - 2*It*N*d*dth^2*m*sin(g1 - th) + GRFy*N*d*l*m*sin(2*g1 - th) - It*N*dg1^2*l*m*sin(2*g1))/(2*m*(It*N*l - Il*d*cos(g1 - th) + Il*N*d*cos(g1 - th)));
        -(GRFx*Il*cos(g1) - GRFy*Il*sin(g1) - GRFx*Il*N*cos(g1) + (Il*dg1^2*m*sin(2*g1))/2 + GRFy*Il*N*sin(g1) + Il*g_reduced*m*sin(g1) + GRFx*l^2*m*cos(g1) - GRFy*l^2*m*sin(g1) + 2*Il*dg1*dl*m + N*l*m*t_rb + N*l*m*t_rf + GRFy*N*l^2*m*sin(g1) - 2*Il*N*dg1*dl*m - Il*d*dth^2*m*sin(g1 - th) - (Il*N*dg1^2*m*sin(2*g1))/2 - (Il*dg1^2*l*m*sin(2*g1))/2 - Il*N*g_reduced*m*sin(g1) - GRFx*N*l^2*m*cos(g1) + GRFx*N*d*l*m*cos(th) - GRFy*N*d*l*m*sin(th) + Il*N*d*dth^2*m*sin(g1 - th) + (Il*N*dg1^2*l*m*sin(2*g1))/2)/(m*(It*N*l - Il*d*cos(g1 - th) + Il*N*d*cos(g1 - th)));
        -(2*GRFx*Il*It*N*cos(g1) - 2*GRFy*Il*It*N*sin(g1) - GRFy*Il*d*m*w*cos(th) - 2*GRFy*Il*d*m_leg*w*cos(th) - GRFx*Il*d*m*w*sin(th) - 2*GRFx*Il*d*m_leg*w*sin(th) + GRFx*Il*N*d^2*m*cos(g1) + 2*Il*N*d*m*t_rb*cos(g1 - th) + 2*Il*N*d*m*t_rf*cos(g1 - th) + 2*GRFx*It*N*l^2*m*cos(g1) - GRFy*Il*N*d^2*m*sin(g1) - 2*GRFy*It*N*l^2*m*sin(g1) + GRFx*Il*N*d^2*m*cos(g1 - 2*th) + 4*Il*It*N*dg1*dl*m + GRFy*Il*N*d^2*m*sin(g1 - 2*th) - 2*Il*d^2*dth^2*m*m_leg*w - GRFy*Il*d*m*w*cos(2*g1 - th) - GRFx*Il*d*m*w*sin(2*g1 - th) + Il*It*N*dg1^2*m*sin(2*g1) + 2*Il*It*N*g_reduced*m*sin(g1) - GRFx*d*l^2*m*m_leg*w*sin(th) - Il*It*N*dg1^2*l*m*sin(2*g1) + Il*d*dg1^2*m*m_leg*w*cos(g1 - th) + 2*GRFy*It*N*l*m*w*cos(g1) + 2*GRFy*It*N*l*m_leg*w*cos(g1) + GRFy*Il*N*d*m*w*cos(th) + 2*GRFy*Il*N*d*m_leg*w*cos(th) + 2*GRFx*It*N*l*m*w*sin(g1) + 2*GRFx*It*N*l*m_leg*w*sin(g1) + GRFx*Il*N*d*m*w*sin(th) + 2*GRFx*Il*N*d*m_leg*w*sin(th) - It*N*dg1^2*l*m*m_leg*w + GRFy*d*l^2*m*m_leg*w*cos(2*g1 - th) + GRFx*d*l^2*m*m_leg*w*sin(2*g1 - th) + 2*Il*d*g_reduced*m*m_leg*w*cos(th) + Il*d*dg1^2*m*m_leg*w*cos(g1 + th) + 2*Il*N*d^2*dth^2*m*m_leg*w - It*N*dg1^2*l^2*m*m_leg*w - 2*Il*It*N*d*dth^2*m*sin(g1 - th) + GRFy*Il*N*d*m*w*cos(2*g1 - th) + GRFx*Il*N*d*m*w*sin(2*g1 - th) - GRFy*d*l^2*m*m_leg*w*cos(th) + It*N*dg1^2*l^2*m*m_leg*w*cos(2*g1) - Il*N*d*dg1^2*m*m_leg*w*cos(g1 + th) - Il*d*dg1^2*l*m*m_leg*w*cos(g1 + th) + 4*Il*d*dg1*dl*m*m_leg*w*sin(g1 - th) + GRFy*N*d^2*l*m*m_leg*w*cos(g1) + GRFy*N*d*l^2*m*m_leg*w*cos(th) + GRFx*N*d^2*l*m*m_leg*w*sin(g1) + 2*N*d*l*m*m_leg*t_rb*w*sin(g1 - th) + 2*N*d*l*m*m_leg*t_rf*w*sin(g1 - th) + GRFx*N*d*l^2*m*m_leg*w*sin(th) - Il*N*d*dg1^2*m*m_leg*w*cos(g1 - th) - GRFy*N*d^2*l*m*m_leg*w*cos(g1 - 2*th) + GRFx*N*d^2*l*m*m_leg*w*sin(g1 - 2*th) + Il*d*dg1^2*l*m*m_leg*w*cos(g1 - th) - It*N*dg1^2*l*m*m_leg*w*cos(2*g1) - GRFy*N*d*l^2*m*m_leg*w*cos(2*g1 - th) - GRFx*N*d*l^2*m*m_leg*w*sin(2*g1 - th) - 2*It*N*g_reduced*l*m*m_leg*w*cos(g1) - 2*Il*N*d*g_reduced*m*m_leg*w*cos(th) + Il*N*d*dg1^2*l*m*m_leg*w*cos(g1 + th) - 4*Il*N*d*dg1*dl*m*m_leg*w*sin(g1 - th) - Il*N*d*dg1^2*l*m*m_leg*w*cos(g1 - th) + 2*It*N*d*dth^2*l*m*m_leg*w*cos(g1 - th))/(4*m*(It*N*l - Il*d*cos(g1 - th) + Il*N*d*cos(g1 - th)));
         (2*GRFy*Il*It*N*sin(g1) - 2*GRFx*Il*It*N*cos(g1) - GRFy*Il*d*m*w*cos(th) - 2*GRFy*Il*d*m_leg*w*cos(th) - GRFx*Il*d*m*w*sin(th) - 2*GRFx*Il*d*m_leg*w*sin(th) - GRFx*Il*N*d^2*m*cos(g1) - 2*Il*N*d*m*t_rb*cos(g1 - th) - 2*Il*N*d*m*t_rf*cos(g1 - th) - 2*GRFx*It*N*l^2*m*cos(g1) + GRFy*Il*N*d^2*m*sin(g1) + 2*GRFy*It*N*l^2*m*sin(g1) - GRFx*Il*N*d^2*m*cos(g1 - 2*th) - 4*Il*It*N*dg1*dl*m - GRFy*Il*N*d^2*m*sin(g1 - 2*th) - 2*Il*d^2*dth^2*m*m_leg*w - GRFy*Il*d*m*w*cos(2*g1 - th) - GRFx*Il*d*m*w*sin(2*g1 - th) - Il*It*N*dg1^2*m*sin(2*g1) - 2*Il*It*N*g_reduced*m*sin(g1) - GRFx*d*l^2*m*m_leg*w*sin(th) + Il*It*N*dg1^2*l*m*sin(2*g1) + Il*d*dg1^2*m*m_leg*w*cos(g1 - th) + 2*GRFy*It*N*l*m*w*cos(g1) + 2*GRFy*It*N*l*m_leg*w*cos(g1) + GRFy*Il*N*d*m*w*cos(th) + 2*GRFy*Il*N*d*m_leg*w*cos(th) + 2*GRFx*It*N*l*m*w*sin(g1) + 2*GRFx*It*N*l*m_leg*w*sin(g1) + GRFx*Il*N*d*m*w*sin(th) + 2*GRFx*Il*N*d*m_leg*w*sin(th) - It*N*dg1^2*l*m*m_leg*w + GRFy*d*l^2*m*m_leg*w*cos(2*g1 - th) + GRFx*d*l^2*m*m_leg*w*sin(2*g1 - th) + 2*Il*d*g_reduced*m*m_leg*w*cos(th) + Il*d*dg1^2*m*m_leg*w*cos(g1 + th) + 2*Il*N*d^2*dth^2*m*m_leg*w - It*N*dg1^2*l^2*m*m_leg*w + 2*Il*It*N*d*dth^2*m*sin(g1 - th) + GRFy*Il*N*d*m*w*cos(2*g1 - th) + GRFx*Il*N*d*m*w*sin(2*g1 - th) - GRFy*d*l^2*m*m_leg*w*cos(th) + It*N*dg1^2*l^2*m*m_leg*w*cos(2*g1) - Il*N*d*dg1^2*m*m_leg*w*cos(g1 + th) - Il*d*dg1^2*l*m*m_leg*w*cos(g1 + th) + 4*Il*d*dg1*dl*m*m_leg*w*sin(g1 - th) + GRFy*N*d^2*l*m*m_leg*w*cos(g1) + GRFy*N*d*l^2*m*m_leg*w*cos(th) + GRFx*N*d^2*l*m*m_leg*w*sin(g1) + 2*N*d*l*m*m_leg*t_rb*w*sin(g1 - th) + 2*N*d*l*m*m_leg*t_rf*w*sin(g1 - th) + GRFx*N*d*l^2*m*m_leg*w*sin(th) - Il*N*d*dg1^2*m*m_leg*w*cos(g1 - th) - GRFy*N*d^2*l*m*m_leg*w*cos(g1 - 2*th) + GRFx*N*d^2*l*m*m_leg*w*sin(g1 - 2*th) + Il*d*dg1^2*l*m*m_leg*w*cos(g1 - th) - It*N*dg1^2*l*m*m_leg*w*cos(2*g1) - GRFy*N*d*l^2*m*m_leg*w*cos(2*g1 - th) - GRFx*N*d*l^2*m*m_leg*w*sin(2*g1 - th) - 2*It*N*g_reduced*l*m*m_leg*w*cos(g1) - 2*Il*N*d*g_reduced*m*m_leg*w*cos(th) + Il*N*d*dg1^2*l*m*m_leg*w*cos(g1 + th) - 4*Il*N*d*dg1*dl*m*m_leg*w*sin(g1 - th) - Il*N*d*dg1^2*l*m*m_leg*w*cos(g1 - th) + 2*It*N*d*dth^2*l*m*m_leg*w*cos(g1 - th))/(4*m*(It*N*l - Il*d*cos(g1 - th) + Il*N*d*cos(g1 - th)))];


end

== matlab function smm_with_grf_tilting_2d/Control/Behavior Control/Primary Leg Behavior/SMM 01/Primary Swing Phase/Leg Trajectory Generator (Normal)/Alpha Target to Leg Length and Leg Angle ==
  data: alpha_v input; dalpha_v input; ddalpha_v input; theta input; dtheta input; l output; dl output; ddl output; phi output; d_y_com parameter; l0_virtual parameter; dphi output; ddphi output
function [l, dl, ddl, phi, dphi, ddphi] = fcn(alpha_v, dalpha_v, ddalpha_v, theta, dtheta, d_y_com, l0_virtual)
    [l, dl, ddl, phi, dphi, ddphi] = AlphaTargetToVirtualLeg2D(alpha_v, dalpha_v, ddalpha_v, theta, dtheta, 0, d_y_com, l0_virtual);
end

== matlab function smm_with_grf_tilting_2d/Control/Behavior Control/Virtual Spring Calculator/Virtual Spring Calculations ==
  data: th input; alpha_v output; dth input; l input; dl input; phi input; dphi input; dalpha_v output; l_v output; dl_v output; d_y_com parameter
function [alpha_v, dalpha_v, l_v, dl_v] = fcn(th, dth, l, dl, phi, dphi, d_y_com)

gma = th + phi;
dgma = dth + dphi;
d = d_y_com;

xf  =  l*sin(gma) - d*sin(th);
dxf =  l*dgma*cos(gma) + dl*sin(gma) - d*dth*cos(th);
yf  = -l*cos(gma) + d*cos(th);
dyf =  l*dgma*sin(gma) - dl*cos(gma) - d*dth*sin(th);

alpha_v  = atan2(yf, xf);
dalpha_v = 1/(1+(yf/xf)^2) * (xf*dyf - yf*dxf)/xf^2;

l_v  = (d^2 + l^2 - 2*d*l*cos(phi))^0.5;
dl_v = (l*dl - d*dl*cos(phi) + d*l*dphi*sin(phi))/l_v;

end

== matlab function smm_with_grf_tilting_2d/Control/Behavior Control/Primary Leg Behavior/SMM 01/Primary Swing Phase/Leg Trajectory Generator (Normal)/Retracted Leg Trajectory ==
  data: start input boolean; t_system input double; t_apex input double; l_apex input double; dl_apex input double; phi_apex input double; dphi_apex input double; l_measured input double; dl_measured input double; phi_measured input double; l output double; dl output double; ddl output double; phi output double; dphi output double; ddphi output double; dphi_measured input double
%% Generates a dynamically feasible trajectory for swinging the virtual leg between two points.
% Constrains to starting/ending positions and velocities.
% Minimizes torque squared
% May want to generate the trajectory in fourbar coordinates instead.
function [l, dl, ddl, phi, dphi, ddphi] = fcn(start, t_system, t_apex, l_apex, dl_apex, phi_apex, dphi_apex, l_measured, dl_measured, phi_measured, dphi_measured)

    persistent t_start l_start phi_start dl_start dphi_start;
    if isempty(t_start)
        t_start = t_system;
        l_start = l_measured;
        dl_start = dl_measured;
        phi_start = phi_measured;
        dphi_start = dphi_measured;
    end
    if start %|| (t_system - t_start) > 0.030
        t_start = t_system;
        l_start = l_measured;
        dl_start = dl_measured;
        phi_start = phi_measured;
        dphi_start = dphi_measured;
    end
    
    t = t_system - t_start;
    time_to_apex = t_apex - t_start;
    t = min(time_to_apex, t);

    % Virtual Leg Length
    [a0, a1, a2, a3] = ThirdOrderTrajectory(l_start, dl_start, l_apex, dl_apex, time_to_apex);
    l = a3*t^3 + a2*t^2 + a1*t + a0;
    dl = 3*a3*t^2 + 2*a2*t + a1;
    ddl = 6*a3*t + 2*a2;
    
    % Virtual Leg Angle
    [a0, a1, a2, a3] = ThirdOrderTrajectory(phi_start, dphi_start, phi_apex, dphi_apex, time_to_apex);
    phi = a3*t^3 + a2*t^2 + a1*t + a0;
    dphi = 3*a3*t^2 + 2*a2*t + a1;
    ddphi = 6*a3*t + 2*a2;

end

== matlab function smm_with_grf_tilting_2d/Control/Behavior Control/Primary Leg Behavior/SMM 01/Primary Swing Phase/Virtual Leg to Four Bar ==
  data: l_leg input; dl_leg input; ddl_leg input; phi input; dphi input; ddphi input; back output; dback output; ddback output; front output; dfront output; ddfront output
function [back, dback, ddback, front, dfront, ddfront] = VirtualLegToFourBar(l_leg, dl_leg, ddl_leg, phi, dphi, ddphi)   
    [back, dback, ddback, front, dfront, ddfront] = VirtualLegToFourBar(l_leg, dl_leg, ddl_leg, phi, dphi, ddphi);
end

== matlab function smm_with_grf_tilting_2d/Control/Behavior Control/Primary Leg Behavior/SMM 01/Primary Swing Phase/Leg Trajectory Generator (Normal)/Avoid Virtual Leg Length Limits1 ==
  data: l_leg_desired input; dl_leg_desired input; ddl_leg_desired input; l_leg_cmd output double; dl_leg_cmd output double; ddl_leg_cmd output double; min_leg_length parameter; max_leg_length parameter
%% Avoid virtual leg length limits by ensuring we don't command position/velocities/accelerations that would hit them.
function [l_leg_cmd, dl_leg_cmd, ddl_leg_cmd] = AvoidVirtualLengthLimits(l_leg_desired, dl_leg_desired, ddl_leg_desired, min_leg_length, max_leg_length)
    [l_leg_cmd, dl_leg_cmd, ddl_leg_cmd] = AvoidVirtualLengthLimits(l_leg_desired, dl_leg_desired, ddl_leg_desired, min_leg_length, max_leg_length);
end
